simulink model "Flipper"  (Simulink 7.9)
settings: Solver=ode45  StartTime=0.0  StopTime=60  RelTol=1e-3
libraries: vrlib x2
settings Model: Creator=karo  LastModifiedBy=karo
settings GRTTargetCC: CombineOutputUpdateFcns=off  GRTInterface=on

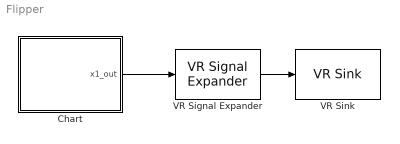
== system Flipper ==
  Chart : Stateflow chart  TreatAsAtomicUnit=on
  VR Signal Expander : vrlib/VR Signal Expander  outwidth=3  outidx=[1 2]
  VR Sink : vrlib/VR Sink  SampleTime=0.05  ViewEnable=on  RemoteChange=off  RemoteView=off  FieldsWritten=Ball.translation.3.1.1.double  WorldFileName=Table.wrl  AutoView=off  VideoDimensions=[]  AllowVariableSize=off
  wires:
  Chart/1(x1_out) -> VR Signal Expander/1
  VR Signal Expander/1 -> VR Sink/1

== stateflow chart Chart ==
  settings: updateMethod=CONTINUOUS
  state Flipper
    during:
    v1_dot = Acc();
    //[v1_dot[0][0], v1_dot[1][0]] = Acc();
    x1_dot = v1;
    // output
    x1_out = x1;
  (default) -> Flipper : {Init();}
  Flipper -> Flipper [order 1] : [HndKontakt() == true]
      | {HndRefl();}
  Flipper -> Flipper [order 4] : [WandUntenKontakt() == true]
      | {WandUntenRefl();}
  Flipper -> Flipper [order 2] : [WandRechtsKontakt() == true]
      | {WandRechtsRefl();}
  Flipper -> Flipper [order 3] : [WandLinksKontakt() == true]
      | {WandLinksRefl();}
  data: a function_output double size=2,1; b function_output boolean; bool function_output boolean; bool function_output boolean; bool function_output boolean; R constant double =0.25; RHnd constant double =0.8; Hnd local double size=2,1; n1 local double size=2,1; n2 local double size=2,1; n3 local double size=2,1; p1 local double size=2,1; p2 local double size=2,1; p3 local double size=2,1; p4 local double size=2,1; t1 local double size=2,1; t2 local double size=2,1; t3 local double size=2,1; v1 local double size=2,1; x1 local double size=2,1; x1_out output double size=2,1
  data v1 settings: updateMethod=SF_CONTINUOUS_TIME_DATA
  data x1 settings: updateMethod=SF_CONTINUOUS_TIME_DATA
  function Init:
    | function Init
    | 
    |     x1 = [4; 5];
    |     v1 = [0; 0];
    |     
    |     Hnd = [6; 2.5];
    |     p1 = [0; 5];
    |     p2 = [5; 0];
    |     p3 = [9; 0];
    |     p4 = [10; 7];
    |     
    |     t1 = (p2 - p1) / norm(p2 - p1);
    |     t2 = (p3 - p2) / norm(p3 - p2);
    |     t3 = (p4 - p3) / norm(p4 - p3);
    |     
    |     n1 = [-t1(2); t1(1)];
    |     n2 = [-t2(2); t2(1)];
    |     n3 = [-t3(2); t3(1)];
  function a = Acc:
    | function a = Acc
    |     a = [0;-1];
    |     %a1 = 0;
    |     %a2 = -1;
    | end
  function b = WandLinksKontakt:
    | function b = WandLinksKontakt
    |     b = false;
    |     
    |     abstand = (x1 - p1)' * n1;  % Abstand von der Achse (p1, p2) in Normalenrichtung
    |     richtung = v1' * n1;        % Bewegungsrichtung der Kugel relativ zu Normalenrichtung
    |     
    |     if ((abstand < R) && (richtung < 0))
    |         b = true;
    |     end
    | end
  function bool = WandUntenKontakt:
    | function bool = WandUntenKontakt
    |     bool = false;
    |     
    |     abstand = (x1 - p2)' * n2;  % Abstand von der Achse (p2, p3) in Normalenrichtung
    |     richtung = v1' * n2;        % Bewegungsrichtung der Kugel relativ zu Normalenrichtung
    |     
    |     if ((abstand < R) && (richtung < 0))
    |         bool = true;
    |     end
    | end
  function bool = WandRechtsKontakt:
    | function bool = WandRechtsKontakt
    |     bool = false;
    |     
    |     abstand = (x1 - p3)' * n3;  % Abstand von der Achse (p3, p4) in Normalenrichtung
    |     richtung = v1' * n3;        % Bewegungsrichtung der Kugel relativ zu Normalenrichtung
    |     
    |     if ((abstand < R) && (richtung < 0))
    |         bool = true;
    |     end
    | end
  function WandLinksRefl:
    | function WandLinksRefl
    |     vt = v1' * t1;
    |     vn = v1' * n1;
    |     
    |     v1 = (vt' * t1) - (vn' * n1);
    | end
  function WandUntenRefl:
    | function WandUntenRefl
    |     vt = v1' * t2;
    |     vn = v1' * n2;
    |     
    |     v1 = (vt' * t2) - (vn' * n2);
    | end
  function WandRechtsRefl:
    | function WandRechtsRefl
    |     vt = v1' * t3;
    |     vn = v1' * n3;
    |     
    |     v1 = (vt' * t3) - (vn' * n3);
    | end
  function bool = HndKontakt:
    | function bool = HndKontakt
    |     bool = false;
    |     
    |     abstand = norm(x1 - Hnd);   % Abstand vom Hindernis
    |     n = (x1 - Hnd) / norm(x1 - Hnd); % Normalenvektor von Hindernis zu Kugel
    |     richtung = v1' * n;        % Bewegungsrichtung der Kugel relativ zu Normalenrichtung
    |     
    |     if ((abstand <= (R + RHnd)) && (richtung < 0))
    |         bool = true;
    |     end
    | end
  function HndRefl:
    | function HndRefl
    |     n = (x1 - Hnd) / norm(x1 - Hnd); % Normalenvektor von Hindernis zu Kugel
    |     t = [n(2); -n(1)];  % Einheitsvektor in Tangentialrichtung
    |     
    |     vt = v1' * t;
    |     vn = v1' * n;
    |     
    |     v1 = (vt' * t) - (vn' * n); % Reflektion
    | end
